simulink model "DroneSimulation"  (R2024a)
settings: Solver=VariableStepAuto  StartTime=0.0  StopTime=100  MaxStep=1e-4  MinStep=1e-6  RelTol=1e-3
undefined symbols (not defined in the file or in its folder): crot, d, g, gustX, gustY, gustZ, I, I_inv, IMU, Ix, Iy, Iz, ks, kt, l, m, ms_mat_inv, pitch_max, rho, roll_max, w_max, windX, windY, windZ, X, Y, Z
libraries: sm_lib x25, nesl_utility x14, simulink x11, slctrl_autotuning x8, mpclib x1, matrix_library x1
(part 3 of 3)

== system DroneSimulation/Controller/xyz control/pitch PID ==
  reference : Inport
  sensor : Inport  Port=2
  Bus Selector2 : BusSelector  OutputSignals=theta,thetaDot
  Clock : Clock  Commented=on
  Closed-Loop PID Autotuner : slctrl_autotuning/Closed-Loop PID Autotuner  Commented=on  PIDType=PID  PIDForm=Parallel  TimeDomain=discrete-time  DiscreteTs=0.1  TuningTs=0.2  UseTuningTs=off  IntegratorFormula=Forward Euler  FilterFormula=Forward Euler  ContinuousTs=0.02  Bandwidth=1  UseExternalWC=off  TargetPM=60  UseExternalPM=off  UseExternalAchievedPM=off  ExperimentMode=Superposition  PlantType=Stable  PlantSign=Positive  AmpSine=1  UseExternalAmpSine=off  UseExternalFRD=off  UseExternalU0=off  UseCompanion=off  NotDeployTuningModule=off  UsePLCCoder=off  OutputMode=control action + perturbation  BlockDataType=double  UseConnectedPID=on  blockpath=[]  tunedP=0  tunedI=0  tunedD=0  tunedN=100  tunedPM=0  EstimationWindowSize=3  UseExternalTuningParams=off  SingleMultiRateVariant=SingleSamplingRate  NumEstimationPeriods=4  NumSettlingPeriods=2  NumOfPRBSPeriod=1  PRBSSignalOrder=12  ExperimentModeVariant=VariantSuperimposed  OutputChoice=VariantCandD
  Compare To Constant : simulink/Logic and Bit Operations/Compare To Constant  Commented=on  relop=<  const=200  OutDataTypeStr=boolean
  Display : Display  Commented=on
  Gain : Gain  Gain=0.5
  Gain1 : Gain  Gain=0.5
  Gain2 : Gain  Gain=0
  Gain3 : Gain  Gain=-1
  Integrator : Integrator
  Sum : Sum  Inputs=|+-
  Sum1 : Sum  Inputs=|+++
  cmd : Outport
  wires:
  Gain2/1 -> Sum1/1
  Bus Selector2/1 -> Closed-Loop PID Autotuner/2, Sum/2  "<theta>"
  sensor/1 -> Bus Selector2/1
  Sum/1 -> Gain/1, Integrator/1
  Gain1/1 -> Sum1/3
  Gain/1 -> Sum1/2
  Integrator/1 -> Gain2/1
  reference/1 -> Sum/1
  Gain3/1 -> Gain1/1
  Clock/1 -> Compare To Constant/1
  Closed-Loop PID Autotuner/3 -> Display/1
  Compare To Constant/1 -> Closed-Loop PID Autotuner/3
  Sum1/1 -> cmd/1, Closed-Loop PID Autotuner/1
  Bus Selector2/2 -> Gain3/1  "<thetaDot>"

== system DroneSimulation/Controller/xyz control/positionController ==
  reference : Inport
  sensor : Inport  Port=2
  Bus Selector : BusSelector  OutputSignals=x,y,psi
  Bus Selector1 : BusSelector  OutputSignals=x,y
  Sum : Sum  Inputs=|+-
  Sum1 : Sum  Inputs=|+-
  pitchPID : Subsystem
  rollPID : Subsystem
  world_to_body : MATLAB Function  TreatAsAtomicUnit=on
  rollRef : Outport
  pitchRef : Outport  Port=2
  wires:
  sensor/1 -> Bus Selector/1
  pitchPID/1(cmd) -> pitchRef/1  "cmd"
  rollPID/1(cmd) -> rollRef/1  "cmd"
  reference/1 -> Bus Selector1/1
  Bus Selector1/1 -> Sum/1  "<x>"
  Bus Selector1/2 -> Sum1/1  "<y>"
  Bus Selector/3 -> world_to_body/3(psi)  "<psi>"
  Bus Selector/2 -> Sum1/2  "<y>"
  Bus Selector/1 -> Sum/2  "<x>"
  Sum1/1 -> world_to_body/2(ey_world)  "ey"
  world_to_body/1(ex_body) -> pitchPID/1(ey)
  world_to_body/2(ey_body) -> rollPID/1(ex)
  Sum/1 -> world_to_body/1(ex_world)  "ex"

== system DroneSimulation/Controller/xyz control/roll PID ==
  reference : Inport
  sensor : Inport  Port=2
  Bus Selector2 : BusSelector  OutputSignals=phi,phiDot
  Clock : Clock  Commented=on
  Closed-Loop PID Autotuner : slctrl_autotuning/Closed-Loop PID Autotuner  Commented=on  PIDType=PID  PIDForm=Parallel  TimeDomain=discrete-time  DiscreteTs=0.1  TuningTs=0.2  UseTuningTs=off  IntegratorFormula=Forward Euler  FilterFormula=Forward Euler  ContinuousTs=0.02  Bandwidth=1  UseExternalWC=off  TargetPM=60  UseExternalPM=off  UseExternalAchievedPM=off  ExperimentMode=Superposition  PlantType=Stable  PlantSign=Positive  AmpSine=1  UseExternalAmpSine=off  UseExternalFRD=off  UseExternalU0=off  UseCompanion=off  NotDeployTuningModule=off  UsePLCCoder=off  OutputMode=control action + perturbation  BlockDataType=double  UseConnectedPID=on  blockpath=[]  tunedP=0  tunedI=0  tunedD=0  tunedN=100  tunedPM=0  EstimationWindowSize=3  UseExternalTuningParams=off  SingleMultiRateVariant=SingleSamplingRate  NumEstimationPeriods=4  NumSettlingPeriods=2  NumOfPRBSPeriod=1  PRBSSignalOrder=12  ExperimentModeVariant=VariantSuperimposed  OutputChoice=VariantCandD
  Compare To Constant : simulink/Logic and Bit Operations/Compare To Constant  Commented=on  relop=<  const=200  OutDataTypeStr=boolean
  Display : Display  Commented=on
  Gain : Gain  Gain=0.5
  Gain1 : Gain  Gain=0.5
  Gain2 : Gain  Gain=0
  Gain3 : Gain  Gain=-1
  Integrator : Integrator
  Sum : Sum  Inputs=|+-
  Sum1 : Sum  Inputs=|+++
  cmd : Outport
  wires:
  Gain2/1 -> Sum1/1
  Bus Selector2/1 -> Sum/2  "<phi>"
  sensor/1 -> Bus Selector2/1
  Bus Selector2/2 -> Gain3/1  "<phiDot>"
  Sum/1 -> Integrator/1, Gain/1
  Gain1/1 -> Sum1/3
  Gain/1 -> Sum1/2
  Integrator/1 -> Gain2/1
  reference/1 -> Sum/1
  Gain3/1 -> Gain1/1
  Compare To Constant/1 -> Closed-Loop PID Autotuner/3
  Clock/1 -> Compare To Constant/1
  Closed-Loop PID Autotuner/3 -> Display/1
  Sum1/1 -> cmd/1, Closed-Loop PID Autotuner/1

== system DroneSimulation/Controller/xyz control/yaw PID ==
  reference : Inport
  sensor : Inport  Port=2
  Bus Selector : BusSelector  OutputSignals=yaw
  Bus Selector2 : BusSelector  OutputSignals=psi,psiDot
  Clock : Clock  Commented=on
  Closed-Loop PID Autotuner : slctrl_autotuning/Closed-Loop PID Autotuner  Commented=on  PIDType=PID  PIDForm=Parallel  TimeDomain=discrete-time  DiscreteTs=0.1  TuningTs=0.2  UseTuningTs=off  IntegratorFormula=Forward Euler  FilterFormula=Forward Euler  ContinuousTs=0.02  Bandwidth=1  UseExternalWC=off  TargetPM=60  UseExternalPM=off  UseExternalAchievedPM=off  ExperimentMode=Superposition  PlantType=Stable  PlantSign=Positive  AmpSine=1  UseExternalAmpSine=off  UseExternalFRD=off  UseExternalU0=off  UseCompanion=off  NotDeployTuningModule=off  UsePLCCoder=off  OutputMode=control action + perturbation  BlockDataType=double  UseConnectedPID=on  blockpath=[]  tunedP=0  tunedI=0  tunedD=0  tunedN=100  tunedPM=0  EstimationWindowSize=3  UseExternalTuningParams=off  SingleMultiRateVariant=SingleSamplingRate  NumEstimationPeriods=4  NumSettlingPeriods=2  NumOfPRBSPeriod=1  PRBSSignalOrder=12  ExperimentModeVariant=VariantSuperimposed  OutputChoice=VariantCandD
  Compare To Constant : simulink/Logic and Bit Operations/Compare To Constant  Commented=on  relop=<  const=200  OutDataTypeStr=boolean
  Display : Display  Commented=on
  Gain : Gain  Gain=0.007688
  Gain1 : Gain  Gain=0.0387
  Gain2 : Gain  Gain=0
  Gain3 : Gain  Gain=-1
  Integrator : Integrator
  Sum : Sum  Inputs=|+-
  Sum1 : Sum  Inputs=|+++
  cmd : Outport
  wires:
  Gain2/1 -> Sum1/1
  Bus Selector2/1 -> Closed-Loop PID Autotuner/2, Sum/2  "<psi>"
  sensor/1 -> Bus Selector2/1
  Gain3/1 -> Gain1/1
  Sum/1 -> Integrator/1, Gain/1
  Gain1/1 -> Sum1/3
  Gain/1 -> Sum1/2
  Integrator/1 -> Gain2/1
  reference/1 -> Bus Selector/1
  Bus Selector/1 -> Sum/1  "<yaw>"
  Compare To Constant/1 -> Closed-Loop PID Autotuner/3
  Clock/1 -> Compare To Constant/1
  Closed-Loop PID Autotuner/3 -> Display/1
  Bus Selector2/2 -> Gain3/1  "<psiDot>"
  Sum1/1 -> cmd/1, Closed-Loop PID Autotuner/1

== system DroneSimulation/DroneModel/Dynamics/ThrustComputation ==
  Angle : Inport
  Fz : Inport  Port=2
  Constant1 : Constant  Value=0
  MatrixMultiply : Product  Multiplication=Matrix(*)
  Mux1 : Mux  Inputs=3
  RotationMatrix : MATLAB Function  TreatAsAtomicUnit=on
  Scope1 : Scope
  Ff : Outport
  wires:
  Constant1/1 -> Mux1/1, Mux1/2
  Fz/1 -> Mux1/3
  RotationMatrix/1(R) -> MatrixMultiply/1
  Mux1/1 -> MatrixMultiply/2  "thrustVector"
  MatrixMultiply/1 -> Scope1/1, Ff/1
  Angle/1 -> RotationMatrix/1(angle)

== system DroneSimulation/DroneModel/Dynamics/rotational aeordynamic drag ==
  omega : Inport
  Constant4 : Constant  Value=crot
  MatrixMultiply3 : Product  Multiplication=Matrix(*)
  Out1 : Outport
  wires:
  Constant4/1 -> MatrixMultiply3/1
  MatrixMultiply3/1 -> Out1/1
  omega/1 -> MatrixMultiply3/2

== system DroneSimulation/Controller/xyz control/positionController/pitchPID ==
  ey : Inport
  Derivative : Derivative
  Gain : Gain  Gain=0.1
  Gain1 : Gain  Gain=0.5
  Gain2 : Gain  Gain=0.001
  Gain3 : Gain
  Integrator : Integrator
  Saturation : Saturate  UpperLimit=pitch_max  LowerLimit=-pitch_max
  Sum1 : Sum  Inputs=|+++
  cmd : Outport
  wires:
  Gain2/1 -> Sum1/1
  Derivative/1 -> Gain1/1
  Gain1/1 -> Sum1/3
  Gain/1 -> Sum1/2
  Integrator/1 -> Gain2/1
  Sum1/1 -> Saturation/1
  Saturation/1 -> Gain3/1
  ey/1 -> Integrator/1, Derivative/1, Gain/1
  Gain3/1 -> cmd/1

== system DroneSimulation/Controller/xyz control/positionController/rollPID ==
  ex : Inport
  Derivative : Derivative
  Gain : Gain  Gain=0.1
  Gain1 : Gain  Gain=0.5
  Gain2 : Gain  Gain=0.001
  Gain3 : Gain  Gain=-1
  Integrator : Integrator
  Saturation : Saturate  UpperLimit=roll_max  LowerLimit=-roll_max
  Sum1 : Sum  Inputs=|+++
  cmd : Outport
  wires:
  Gain2/1 -> Sum1/1
  Derivative/1 -> Gain1/1
  ex/1 -> Integrator/1, Derivative/1, Gain/1
  Gain1/1 -> Sum1/3
  Gain/1 -> Sum1/2
  Integrator/1 -> Gain2/1
  Sum1/1 -> Saturation/1
  Saturation/1 -> Gain3/1
  Gain3/1 -> cmd/1

== matlab function DroneSimulation/Controller/xyz control/positionController/world_to_body ==
  data: ex_world input; ex_body output; ey_world input; psi input; ey_body output
function [ex_body,ey_body] = fcn(ex_world, ey_world, psi)

e_world = [ex_world; ey_world; 0];
%R = [cos(psi) sin(psi); -sin(psi) cos(psi)];

Rinv = [cos(psi), -sin(psi) 0;
      sin(psi), cos(psi), 0;
      0,               0, 1];

e_body = Rinv\e_world;
ex_body = e_body(1);
ey_body = e_body(2);

== matlab function DroneSimulation/DroneModel/Dynamics/ThrustComputation/RotationMatrix ==
  data: angle input; R output
function R = fcn(angle)

phi = angle(1);
theta = angle(2);
psi = angle(3);




% R = [0, 0, cos(psi)*sin(theta)*cos(phi)+sin(phi)*sin(psi);
%      0, 0, sin(psi)*sin(theta)*cos(phi)-cos(psi)*sin(phi);
%      0, 0, cos(theta)*cos(phi)];

% R = [0, 0, -sin(theta)*cos(psi)+sin(phi)*sin(psi);
%      0, 0, -sin(phi)*cos(psi)-sin(theta)*sin(psi);
%      0, 0, cos(theta)];  -> best to now

% 
% R = [cos(phi)*cos(psi) - cos(theta)*sin(phi)*sin(psi),   -cos(psi)*sin(phi)-cos(phi)*cos(theta)*sin(psi), sin(theta)*sin(psi);
%      cos(theta)*cos(psi)*sin(phi) + cos(phi)*sin(psi),   cos(phi)*cos(theta)*cos(psi)-sin(phi)*sin(psi),  -cos(psi)*sin(theta);
%      sin(psi)*sin(theta),                                cos(phi)*sin(theta),                             cos(theta)];

Rz = [cos(psi), -sin(psi) 0;
      sin(psi), cos(psi), 0;
      0,               0, 1];
Ry = [cos(theta), 0, sin(theta);
      0, 1, 0;
      -sin(theta), 0, cos(theta)];
Rx = [1, 0, 0;
      0, cos(phi), -sin(phi);
      0, sin(phi), cos(phi)];

R = Rz*Ry*Rx;



% R = [0 0 ?;
%      0 0 -cos(psi)*sin(theta);
%      0 0 cos(theta)];

== matlab function DroneSimulation/Transmitter/MATLAB Function ==
  data: input input; altitude output; yaw output; altitudeOld input
function [altitude, yaw] = sumRef(input, altitudeOld)

altitude = altitudeOld;
%altitude
if (input == 119) %++
    altitude = altitude + 0.1;
elseif (input==115) %--
    altitude = altitude - 0.1;
end

if (altitude<0)
    altitude = 0;
end

yaw = 0;

== matlab function DroneSimulation/Controller/IMUKalmanFilter/KF ==
  data: IMUmeas input; xhat output; xhat input; P_p input; P_p output
function [xhat, P_p] = fcn(IMUmeas, xhat, P_p)

Q = eye(3)*1e-6;
R = eye(3)*15;
ts = 0.001;  % [s] sampling time

% measurements
w = [IMUmeas(1); IMUmeas(2); IMUmeas(3)];
ax = IMUmeas(4);        % m/s^2
ay = IMUmeas(5);        % m/s^2
az = IMUmeas(6);        % m/s^2

% compute angular accelerations
phi_s = atan2(-ay, abs(az));
theta_s = atan2(ax, abs(az));
psi_s = atan2(ay, ax);
ang = [phi_s; theta_s; psi_s];

P_n = P_p + Q;
K = P_n / (P_n + R);
xkk = xhat + ts.*w;  %model
xhat = xkk + K*(ang - xkk);
P_p = (eye(3)-K)*P_n;

== matlab function DroneSimulation/Sensors/Accelerometer/MATLAB Function ==
  data: phi input; Rinv output; theta input; psi input
function Rinv = fcn(phi, theta, psi)

Rz = [cos(psi), -sin(psi) 0;
      sin(psi), cos(psi), 0;
      0,               0, 1];
Ry = [cos(theta), 0, sin(theta);
      0, 1, 0;
      -sin(theta), 0, cos(theta)];
Rx = [1, 0, 0;
      0, cos(phi), -sin(phi);
      0, sin(phi), cos(phi)];

R = Rz*Ry*Rx;
Rinv = inv(R);
